simulink model "mbd1"  (R2021a)
settings: Solver=FixedStepDiscrete  StartTime=0.0  StopTime=10.0  RelTol=1e-3  EnableMultiTasking=on
libraries: simulink x2
settings Model: Creator=Shereen  LastModifiedBy=Shereen
settings DataIOCC: ReturnWorkspaceOutputs=off
settings OptimizationCC: DefaultParameterBehavior=Inlined  InlineInvariantSignals=on  EnableMemcpy=off  LifeSpan=1  EfficientTunableParamExpr=on
settings DebuggingCC: UnderspecifiedInitializationDetection=Classic  MergeDetectMultiDrivingBlocksExec=none  SFMachineParentedDataDiag=warning  ArithmeticOperatorsInVariantConditions=warning
settings ModelReferenceCC: PropagateSignalLabelsOutOfModel=off
settings SFSimCC: MATLABDynamicMemAlloc=off  CustomCodeUndefinedFunction=UseInterfaceOnly
settings RTWCC: SystemTargetFile=ert.tlc  GenCodeOnly=on  TemplateMakefile=ert_default_tmf  GenerateReport=on  IncludeHyperlinkInReport=on  LaunchReport=on  GenerateTraceInfo=on  GenerateTraceReport=on  GenerateTraceReportSl=on  GenerateTraceReportSf=on  GenerateTraceReportEml=on
settings CodeAppCC: ForceParamTrailComments=on  IgnoreCustomStorageClasses=off  OperatorAnnotations=on  SimulinkDataObjDesc=on  SFDataObjDesc=on  MATLABFcnDesc=on  InsertBlockDesc=on  StateflowObjectComments=on  MATLABSourceComments=on
settings ERTTargetCC: MultiwordLength=2048  GenerateSampleERTMain=on  InlinedParameterPlacement=NonHierarchical  ERTCustomFileTemplate=example_file_process.tlc

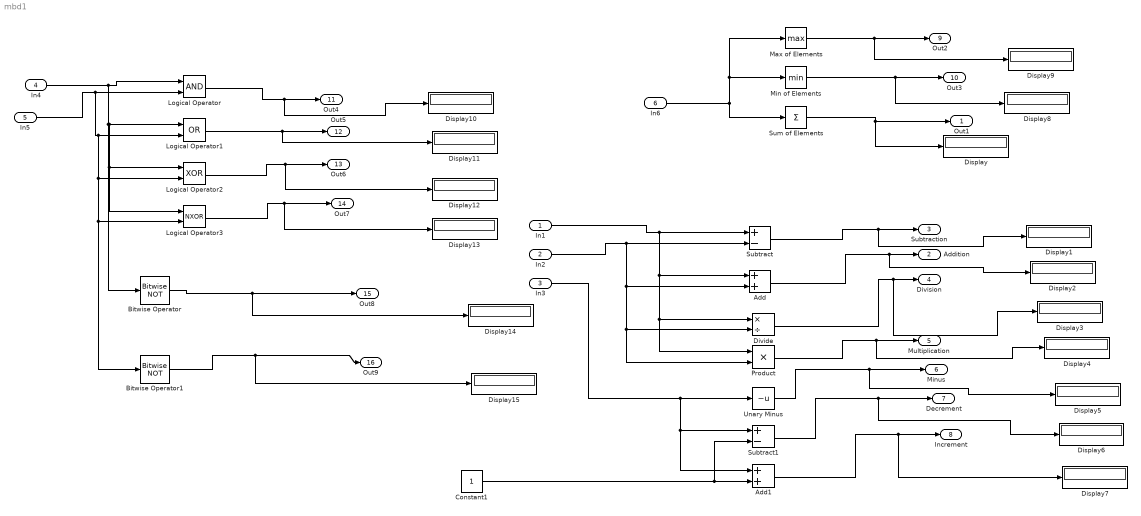
== system mbd1 ==
  In1 : Inport
  In2 : Inport  Port=2
  In3 : Inport  Port=3
  In4 : Inport  Port=4
  In5 : Inport  Port=5
  In6 : Inport  Port=6
  Add : Sum
  Add1 : Sum
  Bitwise Operator : simulink/Logic and Bit Operations/Bitwise Operator  logicop=NOT  UseBitMask=off  BitMask=bin2dec('11011001')  BitMaskRealWorld=Stored Integer
  Bitwise Operator1 : simulink/Logic and Bit Operations/Bitwise Operator  logicop=NOT  UseBitMask=off  BitMask=bin2dec('11011001')  BitMaskRealWorld=Stored Integer
  Constant1 : Constant
  Display{,1..15} (16 alike) : Display
  Divide : Product  Inputs=*/
  Logical Operator : Logic  AllPortsSameDT=off  OutDataTypeStr=boolean
  Logical Operator1 : Logic  Operator=OR  AllPortsSameDT=off  OutDataTypeStr=boolean
  Logical Operator2 : Logic  Operator=XOR  AllPortsSameDT=off  OutDataTypeStr=boolean
  Logical Operator3 : Logic  Operator=NXOR  AllPortsSameDT=off  OutDataTypeStr=boolean
  Max of Elements : MinMax  Function=max
  Min of Elements : MinMax
  Product : Product
  Subtract : Sum  Inputs=+-
  Subtract1 : Sum  Inputs=+-
  Sum of Elements : Sum  Inputs=+
  Unary Minus : UnaryMinus
  Out1 : Outport  SignalName=Sum
  Addition : Outport  Port=2
  Subtraction : Outport  Port=3
  Division : Outport  Port=4
  Multiplication : Outport  Port=5
  Minus : Outport  Port=6
  Decrement : Outport  Port=7
  Increment : Outport  Port=8
  Out2 : Outport  Port=9
  Out3 : Outport  Port=10
  Out4 : Outport  Port=11
  Out5 : Outport  Port=12
  Out6 : Outport  Port=13
  Out7 : Outport  Port=14
  Out8 : Outport  Port=15
  Out9 : Outport  Port=16
  wires:
  Sum of Elements/1 -> Display/1, Out1/1
  In6/1 -> Sum of Elements/1, Min of Elements/1, Max of Elements/1
  Constant1/1 -> Subtract1/2, Add1/2
  In1/1 -> Product/1, Divide/1, Add/1, Subtract/1
  In2/1 -> Product/2, Divide/2, Add/2, Subtract/2
  In3/1 -> Add1/1, Subtract1/1, Unary Minus/1
  Subtract/1 -> Display1/1, Subtraction/1
  Add/1 -> Display2/1, Addition/1
  Divide/1 -> Display3/1, Division/1
  Product/1 -> Display4/1, Multiplication/1
  Add1/1 -> Display7/1, Increment/1
  Subtract1/1 -> Display6/1, Decrement/1
  Unary Minus/1 -> Display5/1, Minus/1
  Max of Elements/1 -> Display9/1, Out2/1
  Min of Elements/1 -> Display8/1, Out3/1
  In4/1 -> Bitwise Operator/1, Logical Operator3/1, Logical Operator2/1, Logical Operator1/1, Logical Operator/1
  In5/1 -> Bitwise Operator1/1, Logical Operator3/2, Logical Operator2/2, Logical Operator1/2, Logical Operator/2
  Logical Operator/1 -> Display10/1, Out4/1
  Logical Operator1/1 -> Display11/1, Out5/1
  Logical Operator2/1 -> Display12/1, Out6/1
  Logical Operator3/1 -> Display13/1, Out7/1
  Bitwise Operator/1 -> Display14/1, Out8/1
  Bitwise Operator1/1 -> Display15/1, Out9/1
